simulink model "GeneratorSystemTestSim"  (R2024a)
settings: Solver=VariableStepAuto  StartTime=0.0  StopTime=10.0  FixedStep=1e-7  RelTol=1e-3
undefined symbols (not defined in the file or in its folder): B, I_gen_max, J, RPM_idle, targetsMCI, tau_gen
libraries: simulink x2, slpidlib x1
settings Model: Creator=henri  LastModifiedBy=henri
settings SolverCC: ZeroCrossAlgorithm=Adaptive
settings DataIOCC: Refine=6
settings DebuggingCC: IgnoredZcDiagnostic=none

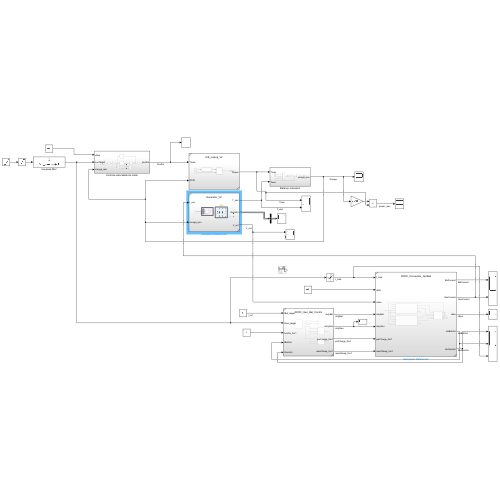
[thumbnail: Simulink's stored preview of the top-level diagram]
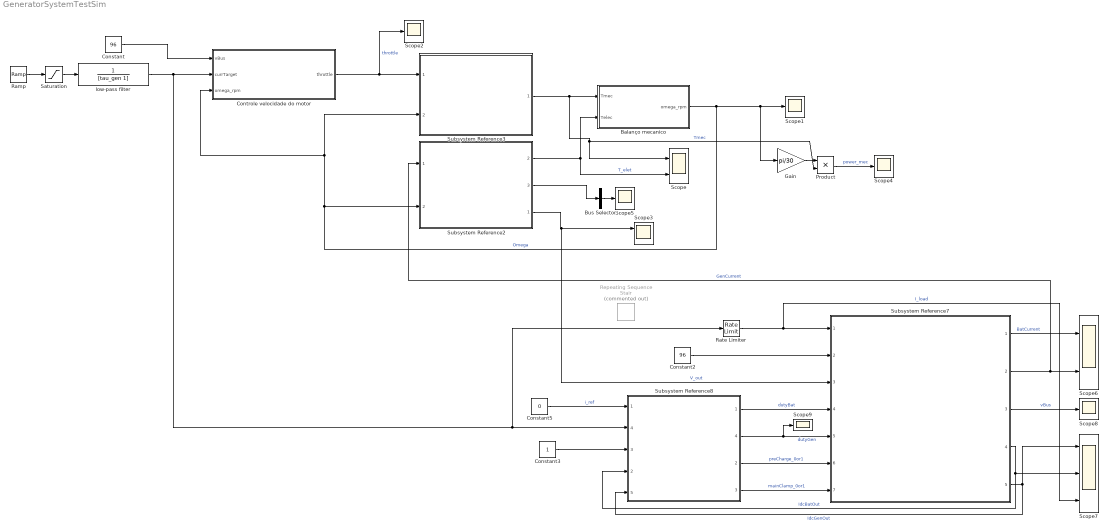
== system GeneratorSystemTestSim ==
  Balanço mecanico : Subsystem
  Bus Selector : BusSelector  OutputSignals=Stator current is_a (A),Stator current is_b (A),Stator current is_c (A)  OutputAsBus=on
  Constant : Constant  Value=96
  Constant2 : Constant  Value=96
  Constant3 : Constant  OutDataTypeStr=boolean
  Constant5 : Constant  Value=0
  Controle velocidade do motor : Subsystem
  Gain : Gain  Gain=pi/30
  Product : Product
  Ramp : simulink/Sources/Ramp  slope=I_gen_max/0.3  start=1  InitialOutput=0
  Rate Limiter : RateLimiter  RisingSlewLimit=100  FallingSlewLimit=-100
  Repeating Sequence Stair : simulink/Sources/Repeating Sequence Stair  Commented=on  OutValues=[0 0.1 10 200 -200].'  tsamp=10  OutMin=[]  OutMax=[]  OutDataTypeStr=double  OutputDataTypeScalingMode=double  OutDataType=fixdt(0,8)  ConRadixGroup=Best Precision: Vector-wise  OutScaling=2^-12
  Saturation : Saturate  UpperLimit=I_gen_max  LowerLimit=0
  Scope : Scope  NumInputPorts=2
  Scope{1..2,4..5,8..9} (6 alike) : Scope
  Scope3 : Scope  NumInputPorts=2
  Scope6 : Scope  NumInputPorts=2
  Scope7 : Scope  NumInputPorts=3
  Subsystem Reference2 : Subsystem  ReferencedSubsystem=Generator_V2
      settings: PortSchema="{\"entries\":[{\"content\":{\"sides\":[{\"content\":{\"connectorIds\":[\"In1\",\"In2\"]},\"type\":\"ConnectorPlacement.EquallySpacedRectSide\",\"uuid\":\"e17fb8a6-b9e2-44fc-9782-17160aaa0541\"},{\"content\":{\"connectorIds\":[\"Out2\",\"Out3\",\"Out1\"],\"side\":\"RIGHT\"},\"type\":\"ConnectorPlacement.EquallySpacedRectSide\",\"uuid\":\"f152f6b9-0348-4082-b4a6-2a28004d56aa\"},{\"content\":{\"side\":\"TOP\"},\"type\":\"ConnectorPlacement.EquallySpacedRectSide\",\"uuid\":\"84bd3409-1ffd-4a2d-b774-99b7aec6f8d1\"}]},\"type\":\"ConnectorPlacement.EquallySpacedConnector\",\"uuid\":\"86673931-c8c4-4310-9ac3-5a0ca8838b0d\"}],\"packageUris\":[\"http://schema.mathworks.com/mf0/Connector/R2020b\"],\"version\":\"1.0\"}"
  Subsystem Reference3 : Subsystem  ReferencedSubsystem=ICE_lookup_V2
  Subsystem Reference7 : Subsystem  ReferencedSubsystem=DCDC_Converters_GenBat
      settings: MinAlgLoopOccurrences=on
  Subsystem Reference8 : Subsystem  ReferencedSubsystem=DCDC_Gen_Bat_Control
      settings: MinAlgLoopOccurrences=on  PortSchema="{\"entries\":[{\"content\":{\"sides\":[{\"content\":{\"connectorIds\":[\"In1\",\"In4\",\"In3\",\"In2\",\"In5\"]},\"type\":\"ConnectorPlacement.EquallySpacedRectSide\",\"uuid\":\"07d7d073-649d-4dd5-ba45-9e0b99c3d986\"},{\"content\":{\"connectorIds\":[\"Out1\",\"Out4\",\"Out2\",\"Out3\"],\"side\":\"RIGHT\"},\"type\":\"ConnectorPlacement.EquallySpacedRectSide\",\"uuid\":\"2b65ab9e-6e2c-411c-94b6-50d3edd52af8\"},{\"content\":{\"side\":\"TOP\"},\"type\":\"ConnectorPlacement.EquallySpacedRectSide\",\"uuid\":\"380bd79d-3c3c-4ed9-b669-43271ad9eab7\"}]},\"type\":\"ConnectorPlacement.EquallySpacedConnector\",\"uuid\":\"a384d7c8-4ab4-46be-9278-b103164c1055\"}],\"packageUris\":[\"http://schema.mathworks.com/mf0/Connector/R2020b\"],\"version\":\"1.0\"}"
  low-pass filter : TransferFcn  Denominator=[tau_gen 1]
  wires:
  Subsystem Reference2/3 -> Bus Selector/1
  Controle velocidade do motor/1(throttle) -> Scope2/1, Subsystem Reference3/1  "throttle"
  Constant/1 -> Controle velocidade do motor/1(vBus)
  Subsystem Reference2/1 -> Subsystem Reference7/3, Scope3/1  "V_out"
  Subsystem Reference3/1 -> Balanço mecanico/1(Tmec), Scope/1, Product/2  "Tmec"
  Balanço mecanico/1(omega_rpm) -> Gain/1, Scope1/1, Subsystem Reference2/2, Subsystem Reference3/2, Controle velocidade do motor/3(omega_rpm)  "Omega"
  Subsystem Reference2/2 -> Balanço mecanico/2(Telec), Scope/2  "T_elet"
  Ramp/1 -> Saturation/1
  Gain/1 -> Product/1
  Product/1 -> Scope4/1  "power_mec"
  Bus Selector/1 -> Scope5/1
  Subsystem Reference7/4 -> Scope7/2, Subsystem Reference8/2  "IdcBatOut"
  Subsystem Reference7/1 -> Scope6/1  "BatCurrent"
  Constant5/1 -> Subsystem Reference8/1  "i_ref"
  Subsystem Reference8/1 -> Subsystem Reference7/4  "dutyBat"
  Constant3/1 -> Subsystem Reference8/3
  Subsystem Reference8/3 -> Subsystem Reference7/7  "mainClamp_0or1"
  Rate Limiter/1 -> Scope7/3, Subsystem Reference7/1  "I_load"
  Subsystem Reference8/2 -> Subsystem Reference7/6  "preCharge_0or1"
  Constant2/1 -> Subsystem Reference7/2
  Subsystem Reference7/2 -> Subsystem Reference2/1, Scope6/2  "GenCurrent"
  Subsystem Reference7/3 -> Scope8/1  "vBus"
  Subsystem Reference7/5 -> Subsystem Reference8/5, Scope7/1  "IdcGenOut"
  Subsystem Reference8/4 -> Scope9/1, Subsystem Reference7/5  "dutyGen"
  low-pass filter/1 -> Rate Limiter/1, Subsystem Reference8/4, Controle velocidade do motor/2(currTarget)
  Saturation/1 -> low-pass filter/1

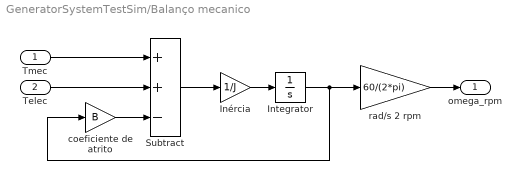
== system GeneratorSystemTestSim/Balanço mecanico ==
  Tmec : Inport
  Telec : Inport  Port=2
  Integrator : Integrator  InitialCondition=RPM_idle*pi/30
  Inércia : Gain  Gain=1/J
  Subtract : Sum  Inputs=++-
  coeficiente de atrito : Gain  Gain=B
  rad/s 2 rpm : Gain  Gain=60/(2*pi)
  omega_rpm : Outport
  wires:
  Integrator/1 -> coeficiente de atrito/1, rad/s 2 rpm/1
  Tmec/1 -> Subtract/1
  Telec/1 -> Subtract/2
  Inércia/1 -> Integrator/1
  Subtract/1 -> Inércia/1
  coeficiente de atrito/1 -> Subtract/3
  rad/s 2 rpm/1 -> omega_rpm/1

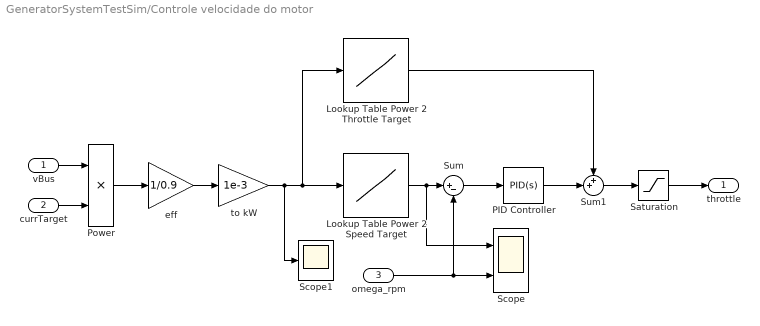
== system GeneratorSystemTestSim/Controle velocidade do motor ==
  vBus : Inport
  currTarget : Inport  Port=2
  omega_rpm : Inport  Port=3
  " Lookup Table Power 2 Speed Target" : Lookup_n-D  NumberOfTableDimensions=1  BreakpointsForDimension1=targetsMCI.Power  Table=targetsMCI.Speed  InternalRulePriority=Speed  RndMeth=Simplest
  " Lookup Table Power 2 Throttle Target" : Lookup_n-D  NumberOfTableDimensions=1  BreakpointsForDimension1=targetsMCI.Power  Table=targetsMCI.Throttle  InternalRulePriority=Speed  RndMeth=Simplest
  PID Controller : slpidlib/PID Controller  Controller=PID  Form=Parallel  TimeDomain=Continuous-time  UseExternalTs=off  SampleTime=-1  IntegratorMethod=Forward Euler  FilterMethod=Forward Euler  ControllerParametersSource=internal  P=0.01  I=0.1  UseKiTs=off  D=0.0001  UseExternalDerivativeSource=off  N=100  UseFilter=on  TunerSelectOption=Transfer Function Based (PID Tuner App)  InitialConditionSource=internal  InitialConditionForIntegrator=0  InitialConditionForFilter=0  DifferentiatorICPrevScaledInput=0  ExternalReset=none  TrackingMode=off  Kt=1  LimitOutput=on  SatLimitsSource=internal  UpperSaturationLimit=90  LowerSaturationLimit=-90  LinearizeAsGain=on  AntiWindupMode=clamping  Kb=1  LimitIntegrator=on  UpperIntegratorSaturationLimit=90  LowerIntegratorSaturationLimit=-90  POutMin=[]  POutMax=[]  IOutMin=[]  IOutMax=[]  DOutMin=[]  DOutMax=[]  NOutMin=[]  NOutMax=[]  SumOutMin=[]  SumOutMax=[]  SaturationOutMin=[]  SaturationOutMax=[]  PParamMin=[]  PParamMax=[]  IParamMin=[]  IParamMax=[]  DParamMin=[]  DParamMax=[]  NParamMin=[]  NParamMax=[]  KbParamMin=[]  KbParamMax=[]  KtParamMin=[]  KtParamMax=[]  KbOutMin=[]  KbOutMax=[]  KtOutMin=[]  KtOutMax=[]  IntegratorOutMin=[]  IntegratorOutMax=[]  FilterOutMin=[]  FilterOutMax=[]  SumI1OutMin=[]  SumI1OutMax=[]  SumI2OutMin=[]  SumI2OutMax=[]  SumI3OutMin=[]  SumI3OutMax=[]  SumI4OutMin=[]  SumI4OutMax=[]  SumDOutMin=[]  SumDOutMax=[]  DifferentiatorOutMin=[]  DifferentiatorOutMax=[]  FilterDiffOutCoefMin=[]  FilterDiffOutCoefMax=[]  ReciprocalOutMin=[]  ReciprocalOutMax=[]  SumDenOutMin=[]  SumDenOutMax=[]  SumNumOutMin=[]  SumNumOutMax=[]  DivideOutMin=[]  DivideOutMax=[]  UdiffTsProdOutMin=[]  UdiffTsProdOutMax=[]  NTsProdOutMin=[]  NTsProdOutMax=[]  UintegralTsProdOutMin=[]  UintegralTsProdOutMax=[]  UngainTsProdOutMin=[]  UngainTsProdOutMax=[]  ClampingZeroOutDataTypeStr=Inherit: Inherit via back propagation  ClampingZeroOutMin=[]  ClampingZeroOutMax=[]  FilterDenConstantOutDataTypeStr=Inherit: Inherit via back propagation  FilterDenConstantOutMin=[]  FilterDenConstantOutMax=[]  PCopyOutDataTypeStr=Inherit: Inherit via back propagation  PCopyOutMin=[]  PCopyOutMax=[]  NCopyOutDataTypeStr=Inherit: Inherit via back propagation  NCopyOutMin=[]  NCopyOutMax=[]  IntegratorContinuousStateAttributes=''  IntegratorStateMustResolveToSignalObject=off  IntegratorRTWStateStorageClass=Auto  FilterContinuousStateAttributes=''  FilterStateMustResolveToSignalObject=off  FilterRTWStateStorageClass=Auto  ParallelPVariant=InternalParameters  IdealPVariant=Disabled  IVariant=InternalParameters  DVariant=InternalParameters  IntegratorVariant=Continuous  SatVariant=Enabled  AWVariant=ContClampingParallel  PCopyVariant=Disabled  TRVariant=Disabled  FdbkBlocksVariant=Forward  IdealPFdbkVariant=Disabled  SatFdbkVariant=Disabled  DerivativeFilterVariant=ContFilter  NVariant=InternalParameters  NCopyVariant=Disabled  FilterICVariant=InternalICsFilter  IntegratorICVariant=InternalICs  ExternalResetVariant=Disabled  TRSumVariant=Passthrough  SumFdbkVariant=Disabled  SumVariant=Sum_PID  TsampFilterVariant=InternalTs  TsampNgainVariant=Passthrough  TsampIntegralVariant=Disabled_SignalSpec  ExternalSaturationOutDataTypeStr=Inherit: Same as second input  DerivativeSourceVariant=ErrorSignal
  Power : Product
  Saturation : Saturate  UpperLimit=90  LowerLimit=5
  Scope : Scope  NumInputPorts=2
  Scope1 : Scope
  Sum : Sum  Inputs=|+-
  Sum1 : Sum  Inputs=++|
  eff : Gain  Gain=1/0.9
  to kW : Gain  Gain=1e-3
  throttle : Outport
  wires:
  omega_rpm/1 -> Scope/2, Sum/2
  Sum/1 -> PID Controller/1
  PID Controller/1 -> Sum1/2
  vBus/1 -> Power/1
  currTarget/1 -> Power/2
  Power/1 -> eff/1
  eff/1 -> to kW/1
  " Lookup Table Power 2 Speed Target"/1 -> Scope/1, Sum/1
  Sum1/1 -> Saturation/1
  " Lookup Table Power 2 Throttle Target"/1 -> Sum1/1
  to kW/1 -> Scope1/1, " Lookup Table Power 2 Throttle Target"/1, " Lookup Table Power 2 Speed Target"/1
  Saturation/1 -> throttle/1
